simulink model "dos_estanques"  (R2023a)
settings: Solver=VariableStepAuto  StartTime=0.0  StopTime=200  RelTol=1e-3
settings Model: Creator=56982  LastModifiedBy=56982
settings SolverCC: AlgebraicLoopSolver=TrustRegion
settings DebuggingCC: UnconnectedInputMsg=warning  UnconnectedOutputMsg=warning  UnconnectedLineMsg=warning
settings ModelReferenceCC: EnableRefExpFcnMdlSchedulingChecks=on

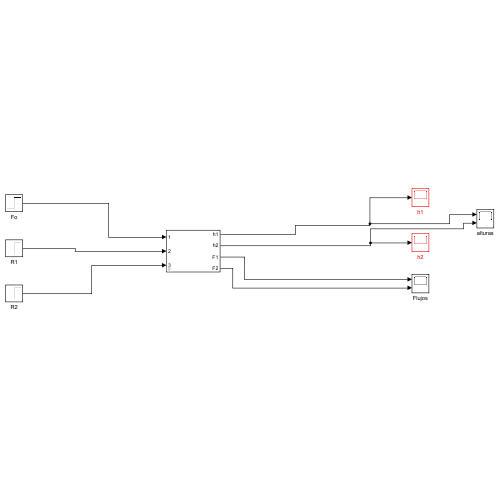
[thumbnail: Simulink's stored preview of the top-level diagram]
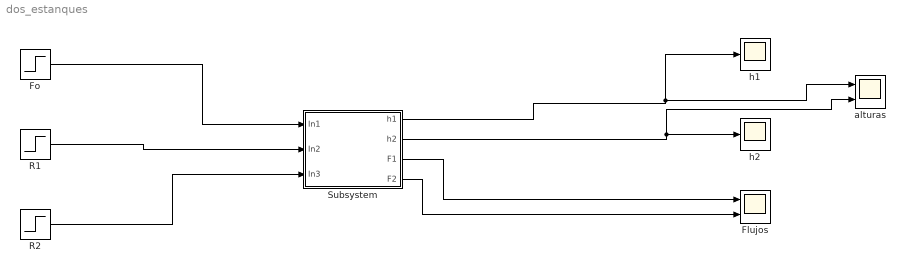
== system dos_estanques ==
  Flujos : Scope  NumInputPorts=2
  Fo : Step  SampleTime=0
  R1 : Step  Time=20  SampleTime=0
  R2 : Step  SampleTime=0
  Subsystem : Subsystem  mask{A1=3, A2=6}
      mask prompts: A1 "Area Estanque 1 (A1):"; A2 "Area Estanque 2 (A2):"
  alturas : Scope  NumInputPorts=2
  h1 : Scope
  h2 : Scope
  wires:
  Fo/1 -> Subsystem/1(In1)
  R1/1 -> Subsystem/2(In2)
  R2/1 -> Subsystem/3(In3)
  Subsystem/1(h1) -> h1/1, alturas/1
  Subsystem/2(h2) -> alturas/2, h2/1
  Subsystem/3(F1) -> Flujos/1
  Subsystem/4(F2) -> Flujos/2

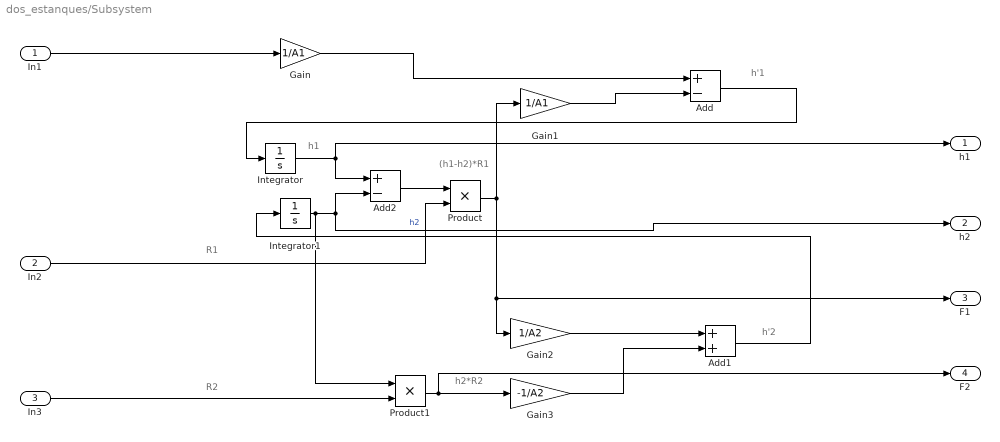
== system dos_estanques/Subsystem ==
  note: R2
  note: (h1-h2)*R1
  note: R1
  note: h2*R2
  note: h1
  note: h'2
  note: h'1
  In1 : Inport
  In2 : Inport  Port=2
  In3 : Inport  Port=3
  Add : Sum  Inputs=+-
  Add1 : Sum
  Add2 : Sum  Inputs=+-
  Gain : Gain  Gain=1/A1
  Gain1 : Gain  Gain=1/A1
  Gain2 : Gain  Gain=1/A2
  Gain3 : Gain  Gain=-1/A2
  Integrator : Integrator
  Integrator1 : Integrator
  Product : Product
  Product1 : Product
  h1 : Outport
  h2 : Outport  Port=2
  F1 : Outport  Port=3
  F2 : Outport  Port=4
  wires:
  Gain1/1 -> Add/2
  Integrator/1 -> h1/1, Add2/1
  Gain2/1 -> Add1/1
  Add/1 -> Integrator/1
  In3/1 -> Product1/2
  Product1/1 -> F2/1, Gain3/1
  Integrator1/1 -> Product1/1, h2/1, Add2/2  "h2"
  Add1/1 -> Integrator1/1
  Product/1 -> F1/1, Gain2/1, Gain1/1
  In2/1 -> Product/2
  Gain/1 -> Add/1
  Gain3/1 -> Add1/2
  Add2/1 -> Product/1
  In1/1 -> Gain/1
